simulink model "PlantWithPressureBus"  (R2023a)
settings: Solver=VariableStepAuto  StartTime=0.0  StopTime=1000000  RelTol=1e-3
settings Model: Creator=alex  LastModifiedBy=alex

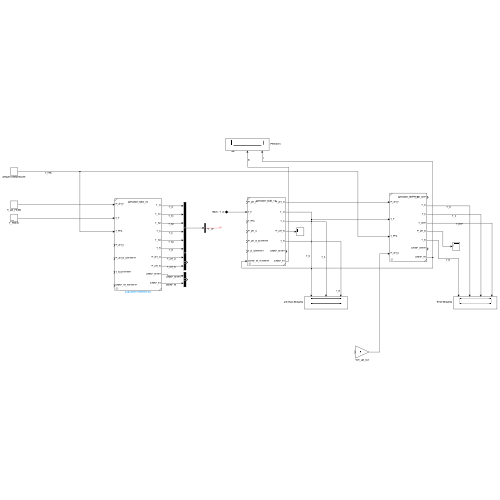
[thumbnail: Simulink's stored preview of the top-level diagram]
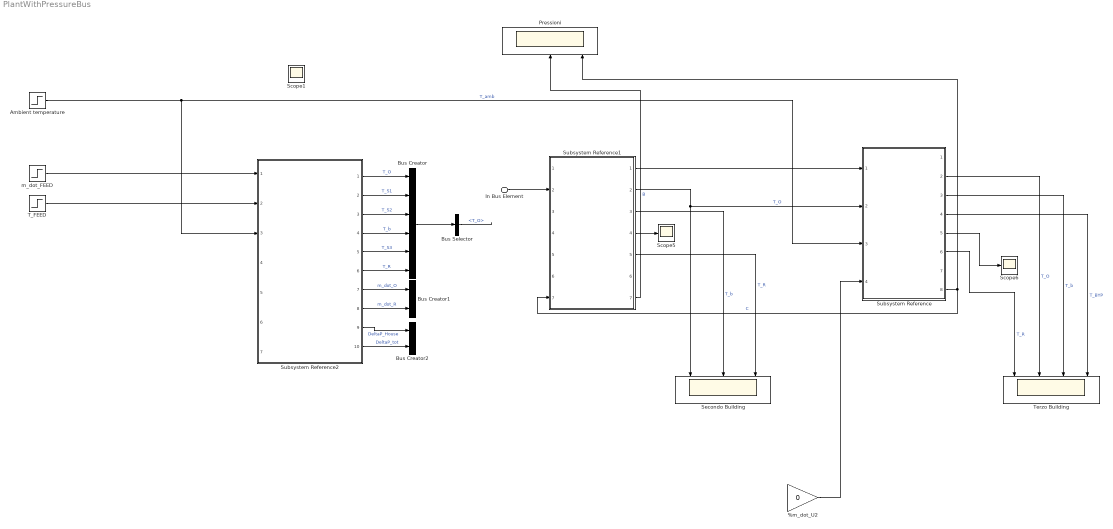
== system PlantWithPressureBus ==
  In Bus Element : Inport  PortName=InBus  Element=T_O
  %m_dot_U2 : Gain  Gain=0
  Ambient temperature : Step  After=300  SampleTime=0
  Bus Creator : BusCreator  Inputs=6
  Bus Creator1 : BusCreator  Inputs=2
  Bus Creator2 : BusCreator  Inputs=2
  Bus Selector : BusSelector  OutputSignals=T_O
  Pressioni : Scope  NumInputPorts=3
  Scope5 : Scope
  Scope6 : Scope
  Secondo Building : Scope  NumInputPorts=3
  Subsystem Reference : Subsystem  ReferencedSubsystem=Simulator_BYP_v3  rho=971  rho_air=971  c_p=4179  c_p_air=4179  pi=3.14151  f_Darcy=0.025  L_F=40.5  D_F=0.4  h_F=1.5  D_S1=0.1  L_S1=5  h_S1=1.5  D_S2=0.025  L_S2=5000  h_S2=300  D_S3=0.1  L_S3=5  h_S3=1.5  D_R=0.4  L_R=40  h_R=1.5  C_b=100  A_b=500  h_b=1.5  D_BYP=0.1  L_BYP=3  h_BYP=1.5  T_F_0=273  T_S1_0=273  T_S2_0=273  T_S3_0=273  T_b_0=273  T_R_0=273
  Subsystem Reference1 : Subsystem  ReferencedSubsystem=Simulator_MID_v3  rho=971  c_p=4179  pi=3.14151  f_Darcy=0.025  L_F=40.5  D_F=0.4  h_F=1.5  D_S1=0.1  L_S1=5  h_S1=1.5  D_S2=0.02  L_S2=50  h_S2=1.5  D_S3=0.1  L_S3=5  h_S3=1.5  D_R=0.4  L_R=40  h_R=1.5  C_b=300  A_b=500  h_b=1.5  T_F_0=273  T_S1_0=273  T_S2_0=273  T_S3_0=273  T_b_0=273  T_R_0=273
  Subsystem Reference2 : Subsystem  ReferencedSubsystem=Simulator_MID_v4  rho=971  c_p=4179  pi=3.14151  f_Darcy=0.025  L_F=40.5  D_F=0.4  h_F=1.5  D_S1=1  L_S1=0.1  h_S1=1.5  D_S2=0.05  L_S2=50  h_S2=1.5  D_S3=0.1  L_S3=5  h_S3=1.5  D_R=0.4  L_R=40  h_R=1.5  C_b=300  A_b=500  h_b=1.5  T_F_0=273  T_S1_0=273  T_S2_0=273  T_S3_0=273  T_b_0=273  T_R_0=273
  T_FEED : Step  Time=0  After=350  SampleTime=0
  Terzo Building : Scope  NumInputPorts=4
  m_dot_FEED : Step  Time=0  After=10  SampleTime=0
  Scope1 : Scope
  wires:
  Subsystem Reference1/1 -> Subsystem Reference/1
  Subsystem Reference1/2 -> Secondo Building/1, Subsystem Reference/2  "T_O"
  Ambient temperature/1 -> Subsystem Reference2/3, Subsystem Reference/3  "T_amb"
  Subsystem Reference/6 -> Terzo Building/1  "T_R"
  Subsystem Reference/5 -> Scope6/1
  %m_dot_U2/1 -> Subsystem Reference/4
  Subsystem Reference/2 -> Terzo Building/2  "T_O"
  Subsystem Reference/3 -> Terzo Building/3  "T_b"
  Subsystem Reference/4 -> Terzo Building/4  "T_BYP"
  Subsystem Reference1/3 -> Secondo Building/2  "T_b"
  Subsystem Reference1/5 -> Secondo Building/3  "T_R"
  Subsystem Reference1/4 -> Scope5/1
  m_dot_FEED/1 -> Subsystem Reference2/1
  T_FEED/1 -> Subsystem Reference2/2
  Subsystem Reference1/7 -> Pressioni/2  "B"
  Subsystem Reference/8 -> Pressioni/3, Subsystem Reference1/7  "C"
  Subsystem Reference2/1 -> Bus Creator/1  "T_O"
  Subsystem Reference2/2 -> Bus Creator/2  "T_S1"
  Subsystem Reference2/3 -> Bus Creator/3  "T_S2"
  Subsystem Reference2/4 -> Bus Creator/4  "T_b"
  Subsystem Reference2/5 -> Bus Creator/5  "T_S3"
  Subsystem Reference2/6 -> Bus Creator/6  "T_R"
  Subsystem Reference2/7 -> Bus Creator1/1  "m_dot_O"
  Subsystem Reference2/8 -> Bus Creator1/2  "m_dot_R"
  Subsystem Reference2/9 -> Bus Creator2/1  "DeltaP_House"
  Subsystem Reference2/10 -> Bus Creator2/2  "DeltaP_tot"
  Bus Creator/1 -> Bus Selector/1
  Bus Selector/1 -> ?  "<T_O>"
  In Bus Element/1 -> Subsystem Reference1/2
